simulink model "SMCDiscreteFinalSim"  (R2024a)
settings: Solver=VariableStepAuto  StartTime=0.0  StopTime=200  RelTol=1e-3
undefined symbols (not defined in the file): a, A_d, B_d, beta, C_d, L_d, T_s
settings Model: Creator=alfar  LastModifiedBy=alfar

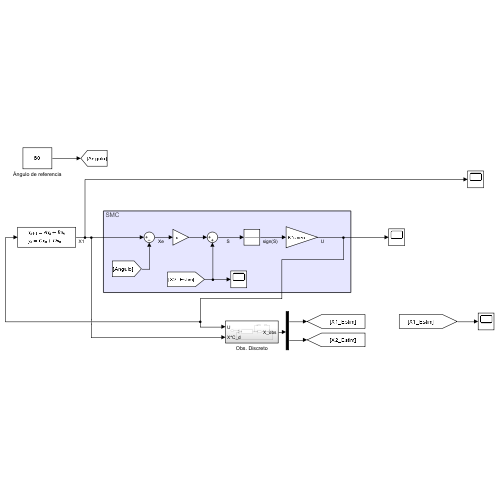
[thumbnail: Simulink's stored preview of the top-level diagram]
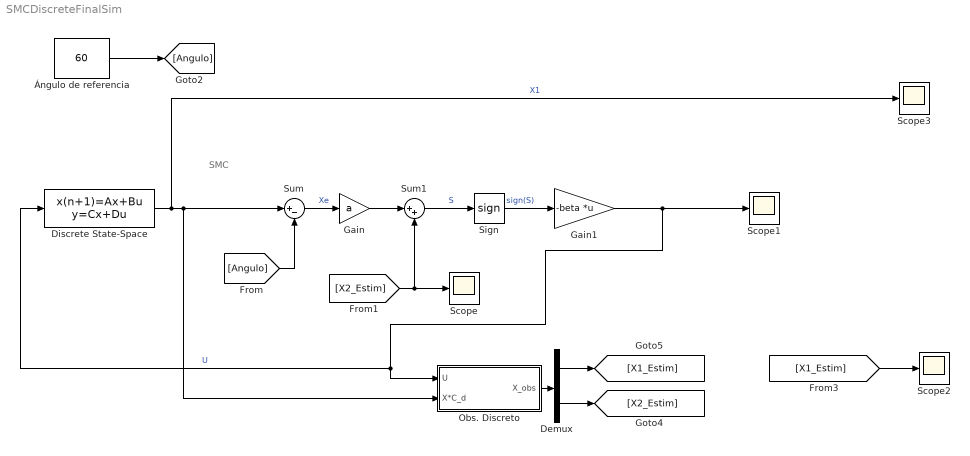
== system SMCDiscreteFinalSim ==
  note: SMC
  Demux : Demux  Outputs=2
  Discrete State-Space : DiscreteStateSpace  A=A_d  B=B_d  C=C_d  D=0  SampleTime=T_s
  Gain : Gain  Gain=a
  Gain1 : Gain  Gain=-beta  Multiplication=Matrix(K*u) (u vector)
  Obs. Discreto : Subsystem
  Scope{,1..3} (4 alike) : Scope
  Sign : Signum  ZeroCross=off
  Sum : Sum  Inputs=|+-
  Sum1 : Sum  Inputs=|++
  Ángulo de referencia : Constant  Value=60
  wires:
  Obs. Discreto/1(X_obs) -> Demux/1
  [X1_Estim] -> Scope2/1
  Demux/2 -> [X2_Estim]
  Gain/1 -> Sum1/1
  [X2_Estim] -> Scope/1, Sum1/2
  [Angulo] -> Sum/2
  Sign/1 -> Gain1/1  "sign(S)"
  Ángulo de referencia/1 -> [Angulo]
  Sum/1 -> Gain/1  "Xe"
  Discrete State-Space/1 -> Scope3/1, Obs. Discreto/2(X*C_d), Sum/1  "X1"
  Sum1/1 -> Sign/1  "S"
  Demux/1 -> [X1_Estim]
  Gain1/1 -> Discrete State-Space/1, Obs. Discreto/1(U), Scope1/1  "U"

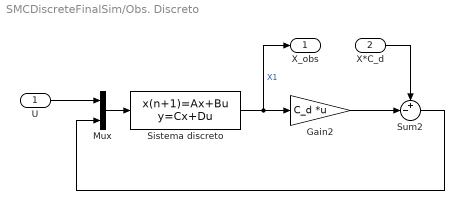
== system SMCDiscreteFinalSim/Obs. Discreto ==
  U : Inport
  X*C_d : Inport  Port=2
  Gain2 : Gain  Gain=C_d  Multiplication=Matrix(K*u)
  Mux : Mux  Inputs=2
  Sistema discreto : DiscreteStateSpace  A=A_d  B=[B_d L_d]  C=eye(2)  D=zeros(2,2)  InitialCondition=[0; 0]  SampleTime=T_s
  Sum2 : Sum  Inputs=+-|
  X_obs : Outport
  wires:
  Gain2/1 -> Sum2/2
  Mux/1 -> Sistema discreto/1
  Sistema discreto/1 -> X_obs/1, Gain2/1  "X1"
  U/1 -> Mux/1
  X*C_d/1 -> Sum2/1
  Sum2/1 -> Mux/2
